simulink model "proxy_linux"  (R2017b)
settings: Solver=ode3  StartTime=0.0  StopTime=inf  FixedStep=0.01  RelTol=1e-3  EnableMultiTasking=on
model workspace (MAT data in the model file):
  SL_ROS_VariableLengthArrays_MaxSizes : struct (value not decoded)
undefined symbols (not defined in the file or in its folder): ampliFactor, ampliFactorDistal, ampliFactorMiddle, filt
libraries: robotlib x11, simulink_extras x11, simulink x8, etargetslib x4, dspnetwork x4
(part 2 of 6)

== system proxy_linux/Generate SchunkCommands /Index Finger/Old Version/Condizionamento ==
  linear_in : Inport
  measure_in : Inport  Port=2
  rotoid_in : Inport  Port=3
  Data Type Conversion : DataTypeConversion  OutDataTypeStr=single
  Display : Display
  Display1 : Display
  Gain Aggiustato : Gain  Gain=50/1000
  Mux : Mux  Inputs=2
  Subsystem : Subsystem
  measure_out : Outport
  sens_out : Outport  Port=2
  wires:
  linear_in/1 -> Gain Aggiustato/1
  Subsystem/1(Deg) -> Display/1
  Gain Aggiustato/1 -> Mux/1
  Data Type Conversion/1 -> measure_out/1
  measure_in/1 -> Data Type Conversion/1
  Subsystem/2(Rad) -> Mux/2, Display1/1
  rotoid_in/1 -> Subsystem/1(Idx Rot)
  Mux/1 -> sens_out/1

== system proxy_linux/Generate SchunkCommands /Index Finger/Old Version/Finger Index  ==
  Mux1 : Mux  Inputs=2
  finger width : Constant  Value=10
  proximal length : Constant  Value=50
  measure : Outport
  wires:
  Mux1/1 -> measure/1
  finger width/1 -> Mux1/1
  proximal length/1 -> Mux1/2

== system proxy_linux/Generate SchunkCommands /Index Finger/Old Version/Pose Generator ==
  "Sensor " : Inport
  measures : Inport  Port=2
  Data Type Conversion Inherited : simulink/Signal Attributes/Data Type Conversion Inherited  ConvertRealWorld=Real World Value  DoSatur=off
      settings: SourceProductName=Simulink  SourceProductBaseCode=SL
  Data Type Conversion Inherited1 : simulink/Signal Attributes/Data Type Conversion Inherited  ConvertRealWorld=Real World Value  DoSatur=off
      settings: SourceProductName=Simulink  SourceProductBaseCode=SL
  Demux : Demux  Outputs=8
  Display : Display
  Display1 : Display
  Jacobian2 : MATLAB Function  TreatAsAtomicUnit=on  SystemSampleTime=0.01
  Pose : MATLAB Function  TreatAsAtomicUnit=on
  Scope : Scope
  Unit Delay1 : UnitDelay  InitialCondition=-1  SampleTime=0.01
  Unit Delay3 : UnitDelay  InitialCondition=[0;2.3]  SampleTime=0.01
  q_0 : Outport
  q_1 : Outport  Port=2
  J : Outport  Port=3
  wires:
  Demux/1 -> Scope/1, q_0/1
  Demux/2 -> q_1/1
  Jacobian2/1(JTcomp) -> J/1, Display/1
  Jacobian2/2(q_next) -> Unit Delay3/1
  Jacobian2/3(J22_ol) -> Unit Delay1/1
  Pose/1(y) -> Display1/1, Jacobian2/1(pose), Demux/1
  measures/1 -> Jacobian2/3(measurements), Pose/2(measurements)
  "Sensor "/1 -> Jacobian2/2(sensor), Pose/1(u)
  Unit Delay1/1 -> Data Type Conversion Inherited/2
  Data Type Conversion Inherited/1 -> Jacobian2/5(J22_old)
  Data Type Conversion Inherited1/1 -> Jacobian2/4(q_pr)
  Unit Delay3/1 -> Data Type Conversion Inherited1/2

== system proxy_linux/Generate SchunkCommands /Middle Finger/Calibration/Subsystem ==
  In1 : Inport
  Enable : EnablePort
  Memory : Memory
  Out1 : Outport
  wires:
  Memory/1 -> Out1/1
  In1/1 -> Memory/1

== system proxy_linux/Generate SchunkCommands /Middle Finger/Calibration1/Subsystem ==
  In1 : Inport
  Enable : EnablePort
  Memory : Memory
  Out1 : Outport
  wires:
  Memory/1 -> Out1/1
  In1/1 -> Memory/1

== system proxy_linux/Generate SchunkCommands /Middle Finger/Subsystem/Subsystem ==
  In1 : Inport
  Enable : EnablePort
  Memory : Memory
  Out1 : Outport
  wires:
  Memory/1 -> Out1/1
  In1/1 -> Memory/1

== system proxy_linux/Generate SchunkCommands /Middle Finger/Subsystem1/Subsystem ==
  In1 : Inport
  Enable : EnablePort
  Memory : Memory
  Out1 : Outport
  wires:
  Memory/1 -> Out1/1
  In1/1 -> Memory/1

== system proxy_linux/Generate SchunkCommands /Ring /calibration/Subsystem ==
  In1 : Inport
  Enable : EnablePort
  Memory : Memory
  Out1 : Outport
  wires:
  Memory/1 -> Out1/1
  In1/1 -> Memory/1

== system proxy_linux/Generate SchunkCommands /Thumb/calibration/Subsystem ==
  In1 : Inport
  Enable : EnablePort
  Memory : Memory
  Out1 : Outport
  wires:
  Memory/1 -> Out1/1
  In1/1 -> Memory/1

== system proxy_linux/Generate SchunkCommands /Thumb/calibration1/Subsystem1 ==
  In1 : Inport
  Enable : EnablePort
  Memory : Memory  InitialCondition=400
  Out1 : Outport
  wires:
  Memory/1 -> Out1/1
  In1/1 -> Memory/1

== system proxy_linux/Generate SchunkCommands /Index Finger/New Version/Condizionamento1/Subsystem ==
  Idx Rot : Inport
  Constant : Constant  Value=2*pi - 20*pi/180 - pi/2  OutDataTypeStr=single
  Gain Vero : Gain  Commented=through  Gain=330/1024
  Gain Aggiustato : Gain  Gain=350*pi/(1024*180)
  Radians to Degrees : simulink_extras/Transformations/Radians to Degrees
  Sum1 : Sum  Inputs=|-+
  Deg : Outport
  Rad : Outport  Port=2
  wires:
  Idx Rot/1 -> Gain Vero/1
  Radians to Degrees/1 -> Deg/1
  Gain Vero/1 -> Gain Aggiustato/1
  Constant/1 -> Sum1/2
  Gain Aggiustato/1 -> Sum1/1
  Sum1/1 -> Radians to Degrees/1, Rad/1

== system proxy_linux/Generate SchunkCommands /Index Finger/Old Version/Condizionamento/Subsystem ==
  Idx Rot : Inport
  Constant : Constant  Value=2*pi - 10*pi/180 - pi/2  OutDataTypeStr=single
  Gain Vero : Gain  Commented=through  Gain=330/1024
  Gain Aggiustato : Gain  Gain=350*pi/(1024*180)
  Radians to Degrees : simulink_extras/Transformations/Radians to Degrees
  Sum1 : Sum  Inputs=|-+
  Deg : Outport
  Rad : Outport  Port=2
  wires:
  Idx Rot/1 -> Gain Vero/1
  Radians to Degrees/1 -> Deg/1
  Gain Vero/1 -> Gain Aggiustato/1
  Constant/1 -> Sum1/2
  Gain Aggiustato/1 -> Sum1/1
  Sum1/1 -> Radians to Degrees/1, Rad/1

== matlab function proxy_linux/Generate SchunkCommands /Finger Spread/MATLAB Function ==
  data: u input; y output; calib input
function y = fcn(u,calib)
%#codegen
y = (-u + calib)/(100);

== matlab function proxy_linux/Generate SchunkCommands /Thumb/MATLAB Function ==
  data: u input; y output
function y = fcn(u)
%#codegen

y = u / 30;

== matlab function proxy_linux/Generate SchunkCommands /Thumb/MATLAB Function1 ==
  data: u input; y output
function y = fcn(u)
%#codegen

y = single( u / 25);

== matlab function proxy_linux/Generate SchunkCommands /Index Finger/New Version/Index New Pose Estimation  ==
  data: Sensors input; pose output; Finger input
function pose = fcn(Sensors, Finger)
%#codegen


lx = Sensors (1);
qB = Sensors (2);

LLM =  Finger(1);   
LIIp = Finger(2);
% LJJp = Finger(3);

% LLM = 50; %fing length
% LIIp = 23.8; %fing width,

%#codegen
LKN = 147.669; %%135.6320;


% LAB =  12.7;
LBC =  43;
LCD =  9;
LDE =  40;
LEF =  27;
LBH =  37; 
LGH =  86;
LGF =  46;
LEJ =  39;
LCI =  16;
% LKL =  24.2;
LKB =  35;
LBK = LKB;
LA2A1 = 13;
LA2B = 16.78;
xL = -10 ;  
offset = 1.8;
yL = - (LIIp - offset);

% LKNx = 134.8;
% LKNy = 15;

% LKLx = -10;
% LKLy = -23;

% qKL = 2.0344;
% qKL = 114.4 * pi / 180; %2.8501;
qKN = 11.5 * pi/180; %%0.1108;

lact = 123; %%117.77;
% lact2 = 13;
% lact3 = 12.5;
% LNO = lact;

LKH = LKB + LBH;

LDF = LDE + LEF;

LBD = LBC + LCD;

LA1N = lx + lact;

LA2K = sqrt(LA2B^2 + LKB^2 - 2*LA2B*LKB*cos(qB));

% qA2
qA2 = my_acos((- LBK^2 + LA2B^2 + LA2K^2)/(2 * LA2B * LA2K));


LA1K = sqrt(LA2A1^2 + LA2K^2 - 2*LA2A1*LA2K*cos(115 * pi/180 - qA2));

    qN = abs(my_acos(((- LA1K^2 + LA1N^2 + LKN^2)/(2*LA1N*LKN)))) - qKN;
    
    xK1 = ((-LA2B^2 + LA2K^2 + LKB^2)/(2*LA2K*LKB));
    
    
    xK2 = (-LA1N^2 + LA1K^2 + LKN^2)/(2*LA1K*LKN);
    xK3 = (-LA2A1^2 + LA2K^2 + LA1K^2)/(2*LA2K*LA1K);
    
    if my_acos(xK1) >= 0
        qK1 = abs(my_acos(xK1));
    else 
        qK1 = abs(my_acos(xK1)) + pi/2;
    end
    
    if my_acos(xK2) >= 0
        qK2 = abs(my_acos(xK2));
    else 
        qK2 = abs(my_acos(xK2)) + pi/2;
    end
    
    if my_acos(xK3) >= 0
        qK3 = abs(my_acos(xK3));
    else 
        qK3 = abs(my_acos(xK3)) + pi/2;
    end
    
        qK = pi - (qK1 + qK2 + qK3 + qKN);
    
xB = - LKB * cos(qK);  yB = LKB * sin(qK);
xH = - LKH * cos(qK);  yH = LKH * sin(qK);
xG = xH - LGH*sin(qK);  yG = yH - LGH*cos(qK);

xC = xB - LBC*cos(qB - qK); yC = yB - LBC * sin(qB - qK);
xD = xC - LCD*cos(qB - qK);   yD = yC - LCD*sin(qB - qK);
xI = xC + LCI * sin(qB - qK);   yI = yC - LCI * cos(qB - qK);

LLI = sqrt((xI - xL)^2 + (yI - yL)^2);

    c1 = sqrt(LLI^2 - LIIp^2);
    
    xj1 = (-LIIp^2 + LLI^2 + c1^2)/(2*c1*LLI);
    
    if my_acos(xj1) >= 0
        qj1 = abs(my_acos(xj1));
    else 
        qj1 = abs(my_acos(xj1)) + pi/2;
    end
    
    qo1 = qj1 + atan((yL - yI)/(xL - xI));



LHD = sqrt((xH - xD)^2 + (yH - yD)^2);

LDG = sqrt((xG - xD)^2 + (yG - yD)^2);


    xG1 = (-LHD^2 + LDG^2 + LGH^2)/(2*LDG*LGH);
    xG2 = (-LDF^2 + LDG^2 + LGF^2)/(2*LDG*LGF);
    
    if my_acos(xG1) >= 0
        qG1 = abs(my_acos(xG1));
    else 
        qG1 = abs(my_acos(xG1)) + pi/2;
    end
    
    if my_acos(xG2) >= 0
        qG2 = abs(my_acos(xG2));
    else 
        qG2 = abs(my_acos(xG2)) + pi/2;
    end

    qG = pi - (qG1 + qG2);
    


xM = xL - LLM*cos(qo1); yM = yL - LLM*sin(qo1);



    xD1 = (-LGH^2 + LHD^2 + LDG^2)/(2*LHD*LDG);
    xD2 = (-LGF^2 + LDG^2 + LDF^2)/(2*LDG*LDF);
    xD3 = (-LBH^2 + LHD^2 + LBD^2)/(2*LHD*LBD);
    
    if my_acos(xD1) >= 0
        qD1 = abs(my_acos(xD1));
    else 
        qD1 = abs(my_acos(xD1)) + pi/2;
    end
    
    if my_acos(xD2) >= 0
        qD2 = abs(my_acos(xD2));
    else 
        qD2 = abs(my_acos(xD2)) + pi/2;
    end

    if my_acos(xD3) >= 0
        qD3 = abs(my_acos(xD3));
    else 
        qD3 = abs(my_acos(xD3)) + pi/2;
    end

    qD = pi - (qD1 + qD2 + qD3);
    
xE = xD - LDE*cos(qB - qD - qK);
yE = yD - LDE*sin(qB - qD - qK);
xJ = xE + LEJ*sin(qB - qD - qK);  
yJ = yE - LEJ*cos(qB - qD - qK);


LJM = sqrt((xJ - xM)^2 + (yJ - yM)^2);

% if LJM^2 - LIIp^2 > 0
    c2 = sqrt(LJM^2 - LIIp^2);
% else
%     c2 = sqrt(-LJM^2 + LIIp^2);
% end

    xj2 = (-LIIp^2 + LJM^2 + c2^2)/(2*c2*LJM);
    
    if my_acos(xj2)>= 0
        qj2 = abs(my_acos(xj2));
    else 
        qj2 = abs(my_acos(xj2)) + pi/2;
    end 
    
    if (xJ - xM)<=0
        qj3 = atan((yJ - yM)/(xJ - xM));
    else
        qj3 = pi + atan((yJ - yM)/(xJ - xM));
    end
    
    qo2 = qj2 + qj3 - qo1;
% if (qo1 < 0)
%     qo1o = jold(1);
% else 
%     qo1o = qo1;
% end
% 
% if (qo2 < 0)
%     qo2o = jold(2);
% else 
%     qo2o = qo2;
% end

    pose = [qo1; qo2; qK; qD; qG; qN; c1; c2 ];
%     dene = [deneK1; deneK2; deneJ1; deneJ2; deneG1; deneG2; deneD1; deneD2; deneD3; deneJ3; deneJ4];
%     
end
%%%
function a = my_acos(b)
    if b < -1
        a = single(-1)
    else
        if b > 1
            a = single(1)
        else
            a = b;
        end
    end
end

== matlab function proxy_linux/Generate SchunkCommands /Index Finger/Old Version/Pose Generator/Pose ==
  data: u input; y output; measurements input
function y  = fcn(u, measurements)
%#codegen
LKN =  135.6320;

LAB =  18;
LBC =  43;
LCD =  9;
LDE =  40;
LEF =  27;
LBH =  37; 
LGH =  86;
LGF =  46;
LEJ =  39;
LCI =  16;
lact = 117.77;
% LNO = lact;

offset = 3;
xL_mag = 10;

LKB =  35;

LKH = LKB + LBH;
LDF = LDE + LEF;
LBD = LBC + LCD;

% LKL =  22.3607;
% LKNx = 134.8;
% LKNy = 15;
% 
% LKLx = -10;
% LKLy = -23;

qKL = 2.0344;
% qKL = 2.8501
% 
%%%%%%%%%%% qKL possibilities
 qKN = 0.1108;
%  qKN = 0.1767;  %% cetvelle olctugume gore cikan aci
% qKN = 0.2653;  %% CAD olcumlerine force sensor farikin ekledigimde cikan aci 


%%%%%%%%%%% finger

% LIIp = 7; %fing width phalange 1
% LJJp = 4; %fing width phalange 2
% LLM =  48;   %fing length
% offset = 3;

LIIp = measurements(1);
LJJp = LIIp;
LLM = measurements(2);


% LIIp = 7;
% LJJp = LIIp;
% LLM = 50;
% offset = 3;
% xL_mag = 10;

% xL = -3;
xL = -xL_mag;  
% xL = -10;
yL = -(LIIp + offset);

lx = u(1);
qB = u(2);

atemp = LAB^2 + LKB^2 - 2*LAB*LKB*cos(qB);
if atemp < 0
    fprintf('errore LAK \n');
    atemp = single(1); % Non 0 se no i denominatori vanno a 0
end
LAK = sqrt(atemp);

if abs((- LAK^2 + (lx+lact)^2 + LKN^2)/(2*(lx+lact)*LKN)) > 1
    fprintf('errore qN');
    qN = single(0);
else
    qN = abs(acos(((- LAK^2 + (lx+lact)^2 + LKN^2)/(2*(lx+lact)*LKN)))) - qKN;
end

xK1 = (-LAB^2 + LAK^2 + LKB^2)/(2*LAK*LKB);
xK2 = (-(lx+lact)^2 + LAK^2 + LKN^2)/(2*LAK*LKN);

%% qK1
if abs(xK1) > 1
    fprintf('errore qK1 \n');
    qK1 = single(0);
else
    if acos(xK1) >= 0
        qK1 = abs(acos(xK1));
    else 
        qK1 = abs(acos(xK1)) + pi/2;
    end
end

%% qK2
if abs(xK2) > 1
    fprintf('errore gK2 \n');
    qK2 = single(0);
else
    if acos(xK2) >= 0
        qK2 = abs(acos(xK2));
    else 
        qK2 = abs(acos(xK2)) + pi/2;
    end
end

    
qK = pi - ( qK1 + qK2 + qKN);
    
xB = - LKB * cos(qK);  yB = LKB * sin(qK);
xH = - LKH * cos(qK);  yH = LKH * sin(qK);
xG = xH - LGH*sin(qK);  yG = yH - LGH*cos(qK);

xC = xB - LBC*cos(qB - qK); yC = yB - LBC * sin(qB - qK);
xD = xC - LCD*cos(qB - qK);   yD = yC - LCD*sin(qB - qK);
xI = xC + LCI * sin(qB - qK);   yI = yC - LCI * cos(qB - qK);

LLI = sqrt((xI - xL)^2 + (yI - yL)^2);
% LLI = 1;

%% c1
atemp = LLI^2 - LIIp^2;
if atemp < 0
    fprintf('errore c1 \n');
    atemp = single(0);
end
c1 = sqrt(atemp);


xj1 = (-LIIp^2 + LLI^2 + c1^2)/(2*c1*LLI);

%% qj1
if abs(xj1) > 1
    fprintf('errore qj1 \n');
    qj1 = single(0);
else
    if acos(xj1) >= 0
        qj1 = abs(acos(xj1));
    else 
        qj1 = abs(acos(xj1)) + pi/2;
    end
end
% qj1 = acos(xj1);
    
qo1_c = qj1 + atan((yL - yI)/(xL - xI));

%%%% SATURATION:
if qo1_c<= 0
    qo1 = abs(qo1_c);
else
    qo1 = qo1_c;
end


    
   
LHD = sqrt((xH - xD)^2 + (yH - yD)^2);
LDG = sqrt((xG - xD)^2 + (yG - yD)^2);
% LHD = 1; LDG = 1;

xG1 = (-LHD^2 + LDG^2 + LGH^2)/(2*LDG*LGH);
xG2 = (-LDF^2 + LDG^2 + LGF^2)/(2*LDG*LGF);

%% qG1
if abs(xG1) > 1
    fprintf('errore qG1 \n')
    qG1 = single(0);
else
    if acos(xG1) >= 0
        qG1 = abs(acos(xG1));
    else 
        qG1 = abs(acos(xG1)) + pi/2;
    end
end

% qG1 = acos(xG1);

%% qG2
if abs(xG2) > 1
    fprintf('errore qG2 \n');
    qG2 = single(0);
else
    if acos(xG2) >= 0
        qG2 = abs(acos(xG2));
    else 
        qG2 = abs(acos(xG2)) + pi/2;
    end
end
% qG2 = acos(xG2);

qG = pi - (qG1 + qG2);

xM = xL - LLM*cos(qo1); yM = yL - LLM*sin(qo1);

xD1 = (-LGH^2 + LHD^2 + LDG^2)/(2*LHD*LDG);
xD2 = (-LGF^2 + LDG^2 + LDF^2)/(2*LDG*LDF);
xD3 = (-LBH^2 + LHD^2 + LBD^2)/(2*LHD*LBD);

%% qD1
if abs(xD1) > 1
    fprintf('errore qD1');
    qD1 = single(0);
else
    if acos(xD1) >= 0
        qD1 = abs(acos(xD1));
    else 
        qD1 = abs(acos(xD1)) + pi/2;
    end
end

%     qD1 = acos(xD1);
%% qD2
if abs(xD2) > 1
    fprintf('errore qD2 \n');
    qD2 = single(0);
else
    if acos(xD2) >= 0
        qD2 = abs(acos(xD2));
    else 
        qD2 = abs(acos(xD2)) + pi/2;
    end
end
% qD2 = acos(xD2);

%% qD3
if abs(xD3) > 1
    fprintf('errore qD3 \n');
    qD3 = single(0);
else
    if acos(xD3) >= 0
        qD3 = abs(acos(xD3));
    else 
        qD3 = abs(acos(xD3)) + pi/2;
    end
end
%     qD3 = acos(xD3);

qD = pi - (qD1 + qD2 + qD3);


xE = xD - LDE*cos(qB - qD - qK);
yE = yD - LDE*sin(qB - qD - qK);
xJ = xE + LEJ*sin(qB - qD - qK);  
yJ = yE - LEJ*cos(qB - qD - qK);

LJM = sqrt((xJ - xM)^2 + (yJ - yM)^2);

atemp = LJM^2 - LJJp^2;
if atemp < 0
    fprintf('errore c2');
    c2 = single(0);
else
    c2 = sqrt(atemp);
end
xj2 = (-LIIp^2 + LJM^2 + c2^2)/(2*c2*LJM);

%% qj2
if abs(xj2) > 1
    fprintf('errore qj2 \n');
    qj2 = single(0);
else
    if acos(xj2) >= 0
        qj2 = abs(acos(xj2));
    else 
        qj2 = abs(acos(xj2)) + pi/2;
    end 
end
% qj2 = acos(xj2);

 if (xJ - xM)<=0
    qj3 = atan((yJ - yM)/(xJ - xM));
else
    qj3 = pi + atan((yJ - yM)/(xJ - xM));
 end


qo2d = qj2 + qj3 - qo1;

if qo2d <= - pi/2
    %Sostituito con la dicitura del codice
    %qo2a = 2*pi + qo2d;
    qo2 = (2*pi + qo2d);% * 0.7;
else 
    %Sostituito con la dicitura del codice
    %qo2a = qo2d; 
    qo2 = (qo2d);% * 0.7; 
end

% 
% if qo2a <= 0
%     qo2 = abs(qo2a);
% else 
%     qo2 = qo2a;
% end


%     if qo2 <= 0
%         qo2 = 0;
%     else if qo2 >= 2.1
%             qo2 = 2.1;
%         else 
%             qo2 = qo2;
%         end
%     end

y = [qo1; qo2; qK; qD; qG; qN; c1; c2];
%     more = [qj2; qj3; xJ - xM; yJ - yM];
%     lengths = [LLM; LIIp];

== matlab function proxy_linux/Generate SchunkCommands /Middle Finger/MATLAB Function2 ==
  data: cons input; sens input; y output; enab input
function y = fcn(cons, sens, enab)

if (enab == 0)
    use = cons;
else 
    use = sens;
end

y = use;

== matlab function proxy_linux/Generate SchunkCommands /Middle Finger/MATLAB Function3 ==
  data: u input; y output; measurements input
function y  = fcn(u, measurements)
%#codegen
LKN =  135.6320;

LAB =  18;
LBC =  43;
LCD =  9;
LDE =  40;
LEF =  27;
LBH =  37; 
LGH =  86;
LGF =  46;
LEJ =  39;
LCI =  16;
lact = 117.77;
% LNO = lact;

offset = 3;
xL_mag = 10;

LKB =  35;

LKH = LKB + LBH;
LDF = LDE + LEF;
LBD = LBC + LCD;

% LKL =  22.3607;
% LKNx = 134.8;
% LKNy = 15;
% 
% LKLx = -10;
% LKLy = -23;

qKL = 2.0344;
% qKL = 2.8501
% 
%%%%%%%%%%% qKL possibilities
 qKN = 0.1108;
%  qKN = 0.1767;  %% cetvelle olctugume gore cikan aci
% qKN = 0.2653;  %% CAD olcumlerine force sensor farikin ekledigimde cikan aci 


%%%%%%%%%%% finger

% LIIp = 7; %fing width phalange 1
% LJJp = 4; %fing width phalange 2
% LLM =  48;   %fing length
% offset = 3;

LIIp = measurements(1);
LJJp = LIIp;
LLM = measurements(2);


% LIIp = 7;
% LJJp = LIIp;
% LLM = 50;
% offset = 3;
% xL_mag = 10;

% xL = -3;
xL = -xL_mag;  
% xL = -10;
yL = -(LIIp + offset);

lx = u(1);
qB = u(2);

atemp = LAB^2 + LKB^2 - 2*LAB*LKB*cos(qB);
if atemp < 0
    fprintf('errore LAK \n');
    atemp = single(1); % Non 0 se no i denominatori vanno a 0
end
LAK = sqrt(atemp);

if abs((- LAK^2 + (lx+lact)^2 + LKN^2)/(2*(lx+lact)*LKN)) > 1
    fprintf('errore qN');
    qN = single(0);
else
    qN = abs(acos(((- LAK^2 + (lx+lact)^2 + LKN^2)/(2*(lx+lact)*LKN)))) - qKN;
end

xK1 = (-LAB^2 + LAK^2 + LKB^2)/(2*LAK*LKB);
xK2 = (-(lx+lact)^2 + LAK^2 + LKN^2)/(2*LAK*LKN);

%% qK1
if abs(xK1) > 1
    fprintf('errore qK1 \n');
    qK1 = single(0);
else
    if acos(xK1) >= 0
        qK1 = abs(acos(xK1));
    else 
        qK1 = abs(acos(xK1)) + pi/2;
    end
end

%% qK2
if abs(xK2) > 1
    fprintf('errore gK2 \n');
    qK2 = single(0);
else
    if acos(xK2) >= 0
        qK2 = abs(acos(xK2));
    else 
        qK2 = abs(acos(xK2)) + pi/2;
    end
end

    
qK = pi - ( qK1 + qK2 + qKN);
    
xB = - LKB * cos(qK);  yB = LKB * sin(qK);
xH = - LKH * cos(qK);  yH = LKH * sin(qK);
xG = xH - LGH*sin(qK);  yG = yH - LGH*cos(qK);

xC = xB - LBC*cos(qB - qK); yC = yB - LBC * sin(qB - qK);
xD = xC - LCD*cos(qB - qK);   yD = yC - LCD*sin(qB - qK);
xI = xC + LCI * sin(qB - qK);   yI = yC - LCI * cos(qB - qK);

LLI = sqrt((xI - xL)^2 + (yI - yL)^2);
% LLI = 1;

%% c1
atemp = LLI^2 - LIIp^2;
if atemp < 0
    fprintf('errore c1 \n');
    atemp = single(0);
end
c1 = sqrt(atemp);


xj1 = (-LIIp^2 + LLI^2 + c1^2)/(2*c1*LLI);

%% qj1
if abs(xj1) > 1
    fprintf('errore qj1 \n');
    qj1 = single(0);
else
    if acos(xj1) >= 0
        qj1 = abs(acos(xj1));
    else 
        qj1 = abs(acos(xj1)) + pi/2;
    end
end
% qj1 = acos(xj1);
    
qo1_c = qj1 + atan((yL - yI)/(xL - xI));

%%%% SATURATION:
if qo1_c<= 0
    qo1 = abs(qo1_c);
else
    qo1 = qo1_c;
end


    
   
LHD = sqrt((xH - xD)^2 + (yH - yD)^2);
LDG = sqrt((xG - xD)^2 + (yG - yD)^2);
% LHD = 1; LDG = 1;

xG1 = (-LHD^2 + LDG^2 + LGH^2)/(2*LDG*LGH);
xG2 = (-LDF^2 + LDG^2 + LGF^2)/(2*LDG*LGF);

%% qG1
if abs(xG1) > 1
    fprintf('errore qG1 \n')
    qG1 = single(0);
else
    if acos(xG1) >= 0
        qG1 = abs(acos(xG1));
    else 
        qG1 = abs(acos(xG1)) + pi/2;
    end
end

% qG1 = acos(xG1);

%% qG2
if abs(xG2) > 1
    fprintf('errore qG2 \n');
    qG2 = single(0);
else
    if acos(xG2) >= 0
        qG2 = abs(acos(xG2));
    else 
        qG2 = abs(acos(xG2)) + pi/2;
    end
end
% qG2 = acos(xG2);

qG = pi - (qG1 + qG2);

xM = xL - LLM*cos(qo1); yM = yL - LLM*sin(qo1);

xD1 = (-LGH^2 + LHD^2 + LDG^2)/(2*LHD*LDG);
xD2 = (-LGF^2 + LDG^2 + LDF^2)/(2*LDG*LDF);
xD3 = (-LBH^2 + LHD^2 + LBD^2)/(2*LHD*LBD);

%% qD1
if abs(xD1) > 1
    fprintf('errore qD1');
    qD1 = single(0);
else
    if acos(xD1) >= 0
        qD1 = abs(acos(xD1));
    else 
        qD1 = abs(acos(xD1)) + pi/2;
    end
end

%     qD1 = acos(xD1);
%% qD2
if abs(xD2) > 1
    fprintf('errore qD2 \n');
    qD2 = single(0);
else
    if acos(xD2) >= 0
        qD2 = abs(acos(xD2));
    else 
        qD2 = abs(acos(xD2)) + pi/2;
    end
end
% qD2 = acos(xD2);

%% qD3
if abs(xD3) > 1
    fprintf('errore qD3 \n');
    qD3 = single(0);
else
    if acos(xD3) >= 0
        qD3 = abs(acos(xD3));
    else 
        qD3 = abs(acos(xD3)) + pi/2;
    end
end
%     qD3 = acos(xD3);

qD = pi - (qD1 + qD2 + qD3);


xE = xD - LDE*cos(qB - qD - qK);
yE = yD - LDE*sin(qB - qD - qK);
xJ = xE + LEJ*sin(qB - qD - qK);  
yJ = yE - LEJ*cos(qB - qD - qK);

LJM = sqrt((xJ - xM)^2 + (yJ - yM)^2);

atemp = LJM^2 - LJJp^2;
if atemp < 0
    fprintf('errore c2');
    c2 = single(0);
else
    c2 = sqrt(atemp);
end
xj2 = (-LIIp^2 + LJM^2 + c2^2)/(2*c2*LJM);

%% qj2
if abs(xj2) > 1
    fprintf('errore qj2 \n');
    qj2 = single(0);
else
    if acos(xj2) >= 0
        qj2 = abs(acos(xj2));
    else 
        qj2 = abs(acos(xj2)) + pi/2;
    end 
end
% qj2 = acos(xj2);

 if (xJ - xM)<=0
    qj3 = atan((yJ - yM)/(xJ - xM));
else
    qj3 = pi + atan((yJ - yM)/(xJ - xM));
 end


qo2d = qj2 + qj3 - qo1;

if qo2d <= - pi/2
    %Sostituito con la dicitura del codice
    %qo2a = 2*pi + qo2d;
    qo2 = (2*pi + qo2d);% * 0.7;
else 
    %Sostituito con la dicitura del codice
    %qo2a = qo2d; 
    qo2 = (qo2d);% * 0.7; 
end

% 
% if qo2a <= 0
%     qo2 = abs(qo2a);
% else 
%     qo2 = qo2a;
% end


%     if qo2 <= 0
%         qo2 = 0;
%     else if qo2 >= 2.1
%             qo2 = 2.1;
%         else 
%             qo2 = qo2;
%         end
%     end

y = [qo1; qo2; qK; qD; qG; qN; c1; c2];
%     more = [qj2; qj3; xJ - xM; yJ - yM];
%     lengths = [LLM; LIIp];
